simulink model "hw6"  (R2021b)
settings: Solver=ode1  StartTime=0.0  StopTime=1e4  FixedStep=0.01  RelTol=1e-3
libraries: simulink x1
settings Model: Creator=A  LastModifiedBy=A

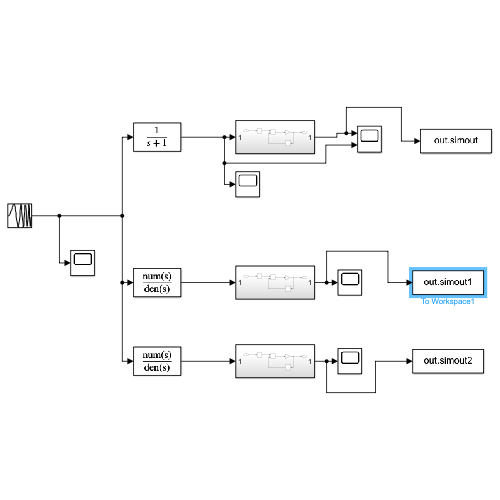
[thumbnail: Simulink's stored preview of the top-level diagram]
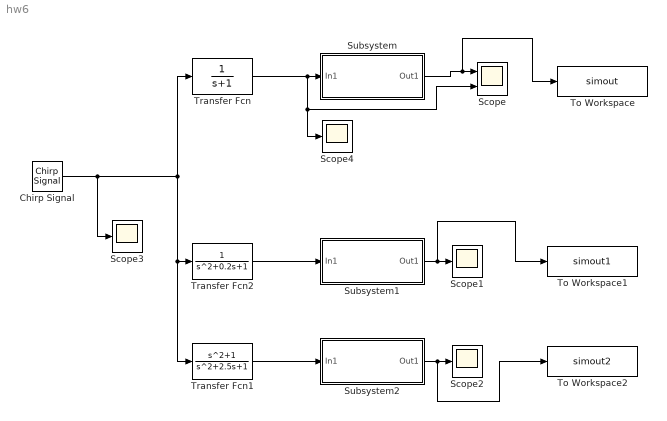
== system hw6 ==
  Chirp Signal : simulink/Sources/Chirp Signal  f1=0.01/(2*pi)  T=1e4  f2=100/(2*pi)
  Scope : Scope  NumInputPorts=2
  Scope{1..4} (4 alike) : Scope
  Subsystem : Subsystem
  Subsystem1 : Subsystem
  Subsystem2 : Subsystem
  To Workspace : ToWorkspace  VariableName=simout  SaveFormat=Timeseries  SampleTime=-1
  To Workspace1 : ToWorkspace  VariableName=simout1  SaveFormat=Timeseries  SampleTime=-1
  To Workspace2 : ToWorkspace  VariableName=simout2  SaveFormat=Timeseries  SampleTime=-1
  Transfer Fcn : TransferFcn  Denominator=[1 1]
  Transfer Fcn1 : TransferFcn  Numerator=[1 0 1]  Denominator=[1 2.5 1]
  Transfer Fcn2 : TransferFcn  Denominator=[1 0.2 1]
  wires:
  Chirp Signal/1 -> Scope3/1, Transfer Fcn2/1, Transfer Fcn1/1, Transfer Fcn/1
  Subsystem/1(Out1) -> To Workspace/1, Scope/1
  Transfer Fcn/1 -> Scope/2, Scope4/1, Subsystem/1(In1)
  Transfer Fcn2/1 -> Subsystem1/1(In1)
  Subsystem1/1(Out1) -> To Workspace1/1, Scope1/1
  Transfer Fcn1/1 -> Subsystem2/1(In1)
  Subsystem2/1(Out1) -> To Workspace2/1, Scope2/1

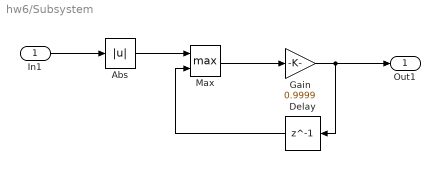
== system hw6/Subsystem ==
  In1 : Inport
  Abs : Abs
  Delay : Delay  DelayLength=1  InitialCondition=1
  Gain : Gain  Gain=0.9999
  Max : MinMax  Function=max  Inputs=2
  Out1 : Outport
  wires:
  Max/1 -> Gain/1
  Gain/1 -> Out1/1, Delay/1
  In1/1 -> Abs/1
  Delay/1 -> Max/2
  Abs/1 -> Max/1

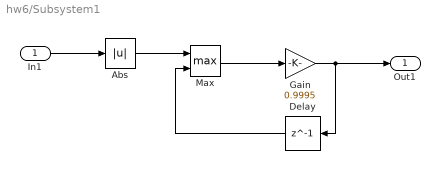
== system hw6/Subsystem1 ==
  In1 : Inport
  Abs : Abs
  Delay : Delay  DelayLength=1  InitialCondition=1
  Gain : Gain  Gain=0.9995
  Max : MinMax  Function=max  Inputs=2
  Out1 : Outport
  wires:
  Max/1 -> Gain/1
  Gain/1 -> Out1/1, Delay/1
  In1/1 -> Abs/1
  Delay/1 -> Max/2
  Abs/1 -> Max/1

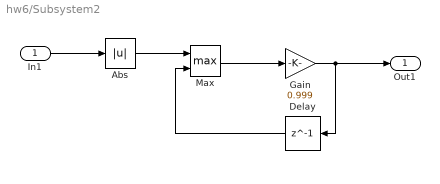
== system hw6/Subsystem2 ==
  In1 : Inport
  Abs : Abs
  Delay : Delay  DelayLength=1  InitialCondition=1
  Gain : Gain  Gain=0.999
  Max : MinMax  Function=max  Inputs=2
  Out1 : Outport
  wires:
  Max/1 -> Gain/1
  Gain/1 -> Out1/1, Delay/1
  In1/1 -> Abs/1
  Delay/1 -> Max/2
  Abs/1 -> Max/1
